simulink model "dut_test"  (R2025b)
settings: Solver=FixedStepDiscrete  StartTime=0.0  StopTime=20.0  RelTol=1e-3
model workspace (MAT data in the model file):
  FL = 8
  WL = 16
settings Model: DataTypeOverride=Off  Creator=Andrei  LastModifiedBy=Andrei
settings SolverCC: AlgebraicLoopSolver=TrustRegion
settings DataIOCC: LimitDataPoints=on  SaveOutput=off  SaveTime=off
settings OptimizationCC: BlockReduction=off  ConditionallyExecuteInputs=off  DefaultParameterBehavior=Inlined  LifeSpan=inf
settings DebuggingCC: AlgebraicLoopMsg=error  SingleTaskRateTransMsg=error  UnconnectedInputMsg=warning  UnconnectedOutputMsg=warning  UnconnectedLineMsg=warning  AllowSymbolicDim=off  StrictBusMsg=ErrorOnBusTreatedAsVector  SFUnexpectedBacktrackingDiag=warning  SFNoUnconditionalDefaultTransitionDiag=warning  SFExecutionAtInitializationDiag=none  ArithmeticOperatorsInVariantConditions=warning
settings HardwareCC: ProdBitPerPointer=32.0  ProdBitPerSizeT=32.0  ProdBitPerPtrDiffT=32.0  ProdLargestAtomicFloat=None  ProdIntDivRoundTo=Undefined  ProdEndianess=Unspecified  ProdWordSize=32.0  ProdHWDeviceType=ASIC/FPGA->ASIC/FPGA  ProdEqTarget=off
settings ModelReferenceCC: EnableRefExpFcnMdlSchedulingChecks=on
settings SFSimCC: SimUseLocalCustomCode=off  CustomCodeUndefinedFunction=UseInterfaceOnly
settings RTWCC: RTWUseLocalCustomCode=off  GPUComputeCapability=3.5
settings CodeAppCC: StateflowObjectComments=on
settings GRTTargetCC: TargetLangStandard=C89/C90 (ANSI)
settings ConfigComp: CovScope=ReferencedModels  CovMetricSettings=dw  CovSaveCumulativeToWorkspaceVar=on  CovSaveSingleToWorkspaceVar=on  CovExternalEMLEnable=off  CovSFcnEnable=off

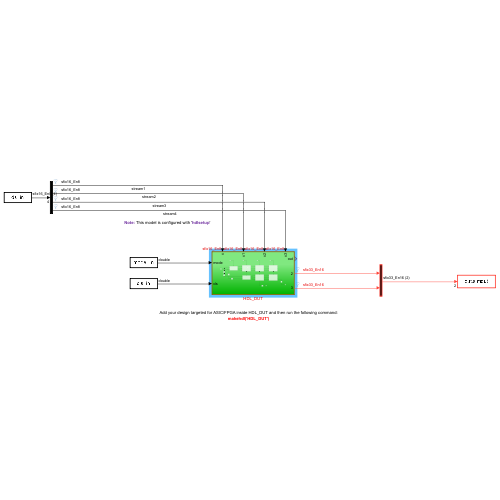
[thumbnail: Simulink's stored preview of the top-level diagram]
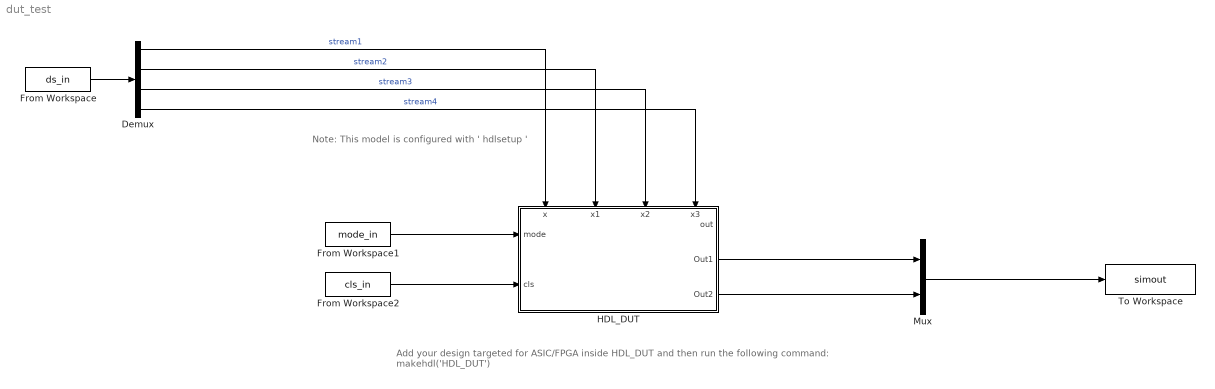
== system dut_test ==
  note: Note: This model is configured with ' hdlsetup '
  note: Add your design targeted for ASIC/FPGA inside HDL_DUT and then run the following command:
      | makehdl('HDL_DUT')
  Demux : Demux
  From Workspace : FromWorkspace  VariableName=ds_in  Interpolate=off  OutputAfterFinalValue=Setting to zero
  From Workspace1 : FromWorkspace  VariableName=mode_in
  From Workspace2 : FromWorkspace  VariableName=cls_in
  HDL_DUT : Subsystem
      settings: PortSchema="{\"entries\":[{\"content\":{\"sides\":[{\"content\":{\"connectorIds\":[\"In1\",\"In2\"]},\"type\":\"ConnectorPlacement.EquallySpacedRectSide\",\"uuid\":\"14bd5ffe-aa4b-486f-999f-3087e859c421\"},{\"content\":{\"connectorIds\":[\"Out1\",\"Out2\",\"Out3\"],\"side\":\"RIGHT\"},\"type\":\"ConnectorPlacement.EquallySpacedRectSide\",\"uuid\":\"689c6885-7600-4ff7-9b81-51456d3620b7\"},{\"content\":{\"connectorIds\":[\"In3\",\"In4\",\"In5\",\"In6\"],\"side\":\"TOP\"},\"type\":\"ConnectorPlacement.EquallySpacedRectSide\",\"uuid\":\"0d9740a3-5156-43d6-94bf-7d829a44bfbd\"}]},\"type\":\"ConnectorPlacement.EquallySpacedConnector\",\"uuid\":\"46e23476-18ad-49d1-a51d-312be1e2c6e8\"}],\"packageUris\":[\"http://schema.mathworks.com/mf0/Connector/R2020b\"],\"version\":\"1.0\"}"
  Mux : Mux  Inputs=2
  To Workspace : ToWorkspace  VariableName=simout  SaveFormat=Timeseries  SampleTime=-1
  wires:
  From Workspace1/1 -> HDL_DUT/1(mode)
  From Workspace2/1 -> HDL_DUT/2(cls)
  Demux/1 -> HDL_DUT/3(x)  "stream1"
  Demux/2 -> HDL_DUT/4(x1)  "stream2"
  Demux/3 -> HDL_DUT/5(x2)  "stream3"
  Demux/4 -> HDL_DUT/6(x3)  "stream4"
  From Workspace/1 -> Demux/1
  HDL_DUT/3(Out2) -> Mux/2
  HDL_DUT/2(Out1) -> Mux/1
  Mux/1 -> To Workspace/1

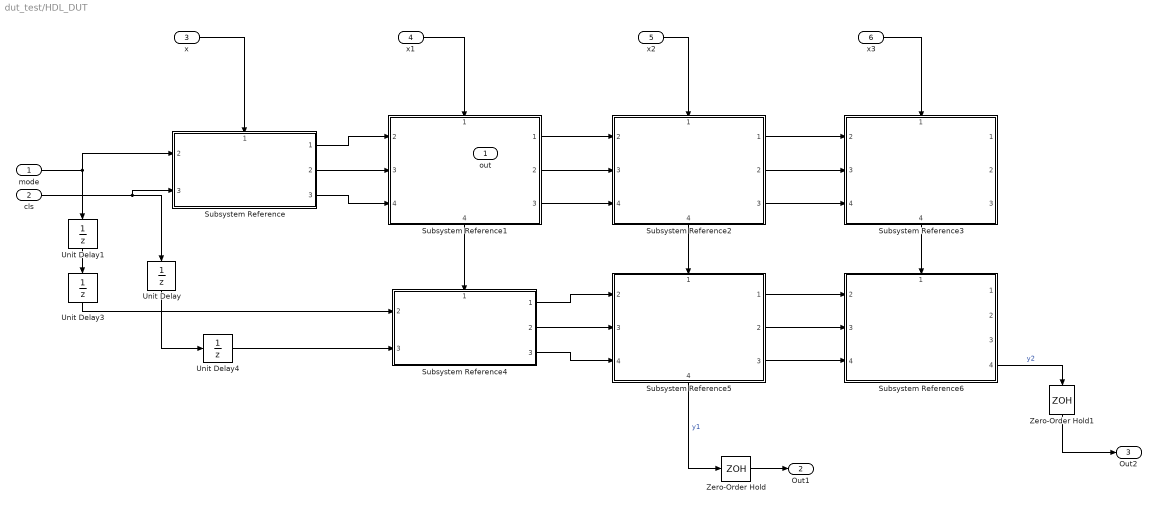
== system dut_test/HDL_DUT ==
  mode : Inport
  cls : Inport  Port=2
  x : Inport  Port=3  OutDataTypeStr=fixdt(1,WL,FL)
  x1 : Inport  Port=4  OutDataTypeStr=fixdt(1,WL,FL)
  x2 : Inport  Port=5  OutDataTypeStr=fixdt(1,WL,FL)
  x3 : Inport  Port=6  OutDataTypeStr=fixdt(1,WL,FL)
  Subsystem Reference : Subsystem  ReferencedSubsystem=boundary_subsys
      settings: PortSchema="{\"entries\":[{\"content\":{\"sides\":[{\"content\":{\"connectorIds\":[\"In2\",\"In3\"]},\"type\":\"ConnectorPlacement.EquallySpacedRectSide\",\"uuid\":\"92a343e4-4510-496d-8069-d6a4c9d6bf12\"},{\"content\":{\"connectorIds\":[\"Out1\",\"Out2\",\"Out3\"],\"side\":\"RIGHT\"},\"type\":\"ConnectorPlacement.EquallySpacedRectSide\",\"uuid\":\"d7c10f84-3430-4177-9926-c1fb8da23e20\"},{\"content\":{\"connectorIds\":[\"In1\"],\"side\":\"TOP\"},\"type\":\"ConnectorPlacement.EquallySpacedRectSide\",\"uuid\":\"976898b3-1521-4361-83a1-553737f64a39\"}]},\"type\":\"ConnectorPlacement.EquallySpacedConnector\",\"uuid\":\"3ce70afe-f04a-487e-8641-2fe6ce8ccb50\"}],\"packageUris\":[\"http://schema.mathworks.com/mf0/Connector/R2020b\"],\"version\":\"1.0\"}"
  Subsystem Reference{1..3,5..6} (5 alike) : Subsystem  ReferencedSubsystem=inner_subsys
      Subsystem Reference1 settings: PortSchema="{\"entries\":[{\"content\":{\"sides\":[{\"content\":{\"connectorIds\":[\"In2\",\"In3\",\"In4\"]},\"type\":\"ConnectorPlacement.EquallySpacedRectSide\",\"uuid\":\"dbc71003-5ddd-4d69-8235-df2a7eac87fb\"},{\"content\":{\"connectorIds\":[\"Out1\",\"Out2\",\"Out3\"],\"side\":\"RIGHT\"},\"type\":\"ConnectorPlacement.EquallySpacedRectSide\",\"uuid\":\"acfb1494-fa6e-460c-affc-491b01631d29\"},{\"content\":{\"connectorIds\":[\"In1\"],\"side\":\"TOP\"},\"type\":\"ConnectorPlacement.EquallySpacedRectSide\",\"uuid\":\"9df206bd-5e7b-487b-8848-9d6785089e3f\"},{\"content\":{\"connectorIds\":[\"Out4\"],\"side\":\"BOTTOM\"},\"type\":\"ConnectorPlacement.EquallySpacedRectSide\",\"uuid\":\"a65c56a2-914f-4631-8a73-1db54343e3c8\"}]},\"type\":\"ConnectorPlacement.EquallySpacedConnector\",\"uuid\":\"2594815e-50bc-4ec3-bffd-73d6907b23c8\"}],\"packageUris\":[\"http://schema.mathworks.com/mf0/Connector/R2020b\"],\"version\":\"1.0\"}"
      Subsystem Reference2 settings: PortSchema="{\"entries\":[{\"content\":{\"sides\":[{\"content\":{\"connectorIds\":[\"In2\",\"In3\",\"In4\"]},\"type\":\"ConnectorPlacement.EquallySpacedRectSide\",\"uuid\":\"dbc71003-5ddd-4d69-8235-df2a7eac87fb\"},{\"content\":{\"connectorIds\":[\"Out1\",\"Out2\",\"Out3\"],\"side\":\"RIGHT\"},\"type\":\"ConnectorPlacement.EquallySpacedRectSide\",\"uuid\":\"acfb1494-fa6e-460c-affc-491b01631d29\"},{\"content\":{\"connectorIds\":[\"In1\"],\"side\":\"TOP\"},\"type\":\"ConnectorPlacement.EquallySpacedRectSide\",\"uuid\":\"9df206bd-5e7b-487b-8848-9d6785089e3f\"},{\"content\":{\"connectorIds\":[\"Out4\"],\"side\":\"BOTTOM\"},\"type\":\"ConnectorPlacement.EquallySpacedRectSide\",\"uuid\":\"8966e87e-b0a8-4cc4-bc92-71ad54fbd042\"}]},\"type\":\"ConnectorPlacement.EquallySpacedConnector\",\"uuid\":\"2594815e-50bc-4ec3-bffd-73d6907b23c8\"}],\"packageUris\":[\"http://schema.mathworks.com/mf0/Connector/R2020b\"],\"version\":\"1.0\"}"
      Subsystem Reference3 settings: PortSchema="{\"entries\":[{\"content\":{\"sides\":[{\"content\":{\"connectorIds\":[\"In2\",\"In3\",\"In4\"]},\"type\":\"ConnectorPlacement.EquallySpacedRectSide\",\"uuid\":\"dbc71003-5ddd-4d69-8235-df2a7eac87fb\"},{\"content\":{\"connectorIds\":[\"Out1\",\"Out2\",\"Out3\"],\"side\":\"RIGHT\"},\"type\":\"ConnectorPlacement.EquallySpacedRectSide\",\"uuid\":\"acfb1494-fa6e-460c-affc-491b01631d29\"},{\"content\":{\"connectorIds\":[\"In1\"],\"side\":\"TOP\"},\"type\":\"ConnectorPlacement.EquallySpacedRectSide\",\"uuid\":\"9df206bd-5e7b-487b-8848-9d6785089e3f\"},{\"content\":{\"connectorIds\":[\"Out4\"],\"side\":\"BOTTOM\"},\"type\":\"ConnectorPlacement.EquallySpacedRectSide\",\"uuid\":\"2e8e6e29-b6f8-437f-8718-04defcb9d1be\"}]},\"type\":\"ConnectorPlacement.EquallySpacedConnector\",\"uuid\":\"2594815e-50bc-4ec3-bffd-73d6907b23c8\"}],\"packageUris\":[\"http://schema.mathworks.com/mf0/Connector/R2020b\"],\"version\":\"1.0\"}"
      Subsystem Reference5 settings: PortSchema="{\"entries\":[{\"content\":{\"sides\":[{\"content\":{\"connectorIds\":[\"In2\",\"In3\",\"In4\"]},\"type\":\"ConnectorPlacement.EquallySpacedRectSide\",\"uuid\":\"dbc71003-5ddd-4d69-8235-df2a7eac87fb\"},{\"content\":{\"connectorIds\":[\"Out1\",\"Out2\",\"Out3\"],\"side\":\"RIGHT\"},\"type\":\"ConnectorPlacement.EquallySpacedRectSide\",\"uuid\":\"acfb1494-fa6e-460c-affc-491b01631d29\"},{\"content\":{\"connectorIds\":[\"In1\"],\"side\":\"TOP\"},\"type\":\"ConnectorPlacement.EquallySpacedRectSide\",\"uuid\":\"9df206bd-5e7b-487b-8848-9d6785089e3f\"},{\"content\":{\"connectorIds\":[\"Out4\"],\"side\":\"BOTTOM\"},\"type\":\"ConnectorPlacement.EquallySpacedRectSide\",\"uuid\":\"f5ac06d2-d4e5-4499-bb33-6140b0a1c1fa\"}]},\"type\":\"ConnectorPlacement.EquallySpacedConnector\",\"uuid\":\"2594815e-50bc-4ec3-bffd-73d6907b23c8\"}],\"packageUris\":[\"http://schema.mathworks.com/mf0/Connector/R2020b\"],\"version\":\"1.0\"}"
      Subsystem Reference6 settings: PortSchema="{\"entries\":[{\"content\":{\"sides\":[{\"content\":{\"connectorIds\":[\"In2\",\"In3\",\"In4\"]},\"type\":\"ConnectorPlacement.EquallySpacedRectSide\",\"uuid\":\"dbc71003-5ddd-4d69-8235-df2a7eac87fb\"},{\"content\":{\"connectorIds\":[\"Out1\",\"Out2\",\"Out3\",\"Out4\"],\"side\":\"RIGHT\"},\"type\":\"ConnectorPlacement.EquallySpacedRectSide\",\"uuid\":\"acfb1494-fa6e-460c-affc-491b01631d29\"},{\"content\":{\"connectorIds\":[\"In1\"],\"side\":\"TOP\"},\"type\":\"ConnectorPlacement.EquallySpacedRectSide\",\"uuid\":\"9df206bd-5e7b-487b-8848-9d6785089e3f\"}]},\"type\":\"ConnectorPlacement.EquallySpacedConnector\",\"uuid\":\"2594815e-50bc-4ec3-bffd-73d6907b23c8\"}],\"packageUris\":[\"http://schema.mathworks.com/mf0/Connector/R2020b\"],\"version\":\"1.0\"}"
  Subsystem Reference4 : Subsystem  ReferencedSubsystem=boundary_subsys
      settings: PortSchema="{\"entries\":[{\"content\":{\"sides\":[{\"content\":{\"connectorIds\":[\"In2\",\"In3\"]},\"type\":\"ConnectorPlacement.EquallySpacedRectSide\",\"uuid\":\"92a343e4-4510-496d-8069-d6a4c9d6bf12\"},{\"content\":{\"connectorIds\":[\"Out1\",\"Out2\",\"Out3\"],\"side\":\"RIGHT\"},\"type\":\"ConnectorPlacement.EquallySpacedRectSide\",\"uuid\":\"d7c10f84-3430-4177-9926-c1fb8da23e20\"},{\"content\":{\"connectorIds\":[\"In1\"],\"side\":\"TOP\"},\"type\":\"ConnectorPlacement.EquallySpacedRectSide\",\"uuid\":\"976898b3-1521-4361-83a1-553737f64a39\"}]},\"type\":\"ConnectorPlacement.EquallySpacedConnector\",\"uuid\":\"3ce70afe-f04a-487e-8641-2fe6ce8ccb50\"}],\"packageUris\":[\"http://schema.mathworks.com/mf0/Connector/R2020b\"],\"version\":\"1.0\"}"
  Unit Delay{,1,3..4} (4 alike) : UnitDelay  SampleTime=-1  HasFrameUpgradeWarning=on
  Zero-Order Hold : ZeroOrderHold
  Zero-Order Hold1 : ZeroOrderHold
  out : Outport  VectorParamsAs1DForOutWhenUnconnected=off
  Out1 : Outport  Port=2
  Out2 : Outport  Port=3
  wires:
  x/1 -> Subsystem Reference/1
  x3/1 -> Subsystem Reference3/1
  x2/1 -> Subsystem Reference2/1
  Subsystem Reference2/4 -> Subsystem Reference5/1
  Subsystem Reference4/2 -> Subsystem Reference5/3
  Subsystem Reference4/1 -> Subsystem Reference5/2
  Subsystem Reference5/2 -> Subsystem Reference6/3
  Subsystem Reference5/1 -> Subsystem Reference6/2
  Subsystem Reference1/4 -> Subsystem Reference4/1
  Subsystem Reference4/3 -> Subsystem Reference5/4
  Unit Delay1/1 -> Unit Delay3/1
  Subsystem Reference1/3 -> Subsystem Reference2/4
  Subsystem Reference2/1 -> Subsystem Reference3/2
  mode/1 -> Unit Delay1/1, Subsystem Reference/2
  Subsystem Reference/3 -> Subsystem Reference1/4
  Subsystem Reference/1 -> Subsystem Reference1/2
  Unit Delay/1 -> Unit Delay4/1
  Subsystem Reference2/3 -> Subsystem Reference3/4
  Subsystem Reference5/3 -> Subsystem Reference6/4
  Subsystem Reference/2 -> Subsystem Reference1/3
  cls/1 -> Unit Delay/1, Subsystem Reference/3
  Subsystem Reference1/2 -> Subsystem Reference2/3
  Subsystem Reference5/4 -> Zero-Order Hold/1  "y1"
  Subsystem Reference2/2 -> Subsystem Reference3/3
  Subsystem Reference1/1 -> Subsystem Reference2/2
  Subsystem Reference3/4 -> Subsystem Reference6/1
  Subsystem Reference6/4 -> Zero-Order Hold1/1  "y2"
  x1/1 -> Subsystem Reference1/1
  Unit Delay3/1 -> Subsystem Reference4/2
  Unit Delay4/1 -> Subsystem Reference4/3
  Zero-Order Hold/1 -> Out1/1
  Zero-Order Hold1/1 -> Out2/1
